simulink model "PIDPlus_1"  (R2023b)
settings: Solver=VariableStepAuto  StartTime=0.0  StopTime=50  RelTol=1e-3
undefined symbols (not defined in the file): Kd, Ki, Kp, Treset
settings Model: Creator=CANER  LastModifiedBy=CANER

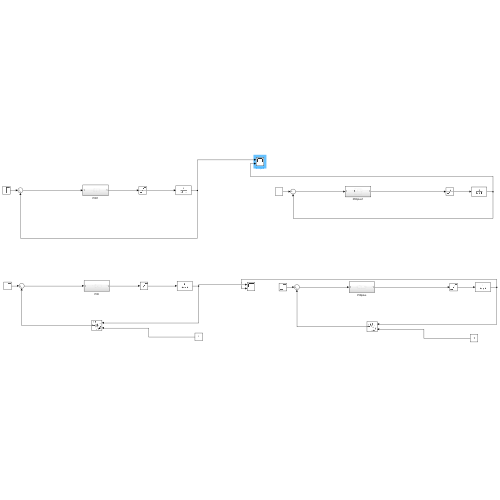
[thumbnail: Simulink's stored preview of the top-level diagram]
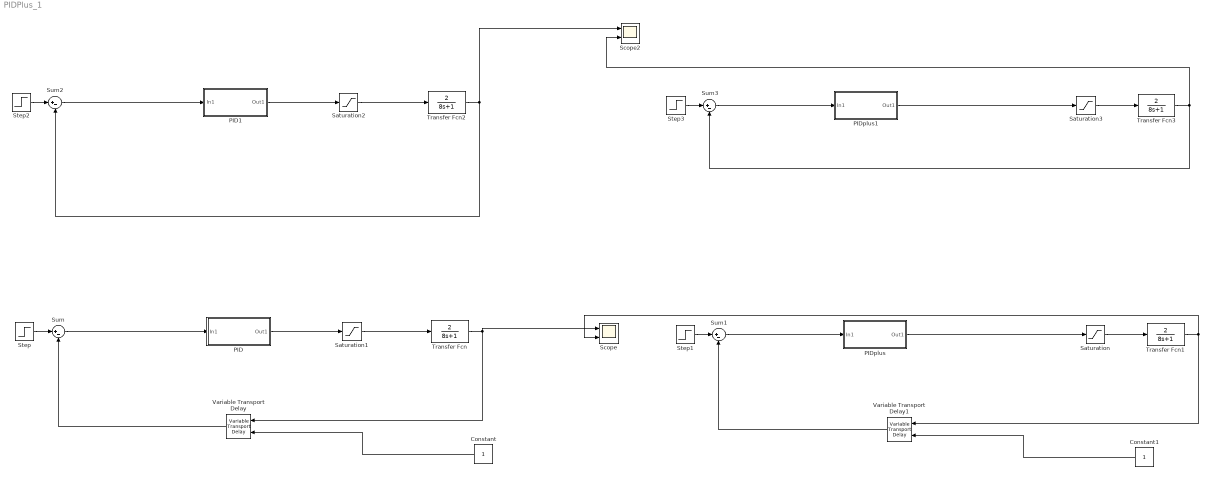
== system PIDPlus_1 ==
  Constant : Constant
  Constant1 : Constant
  PID : Subsystem
  PID1 : Subsystem
  PIDplus : Subsystem
  PIDplus1 : Subsystem
  Saturation{,1..3} (4 alike) : Saturate
  Scope : Scope  NumInputPorts=2
  Scope2 : Scope  NumInputPorts=2
  Step{,1..3} (4 alike) : Step  SampleTime=0
  Sum{,1..3} (4 alike) : Sum  Inputs=|+-
  Transfer Fcn{,1..3} (4 alike) : TransferFcn  Numerator=[2]  Denominator=[8 1]
  Variable Transport Delay : VariableTransportDelay  VariableDelayType=Variable transport delay  MaximumDelay=10
  Variable Transport Delay1 : VariableTransportDelay  VariableDelayType=Variable transport delay  MaximumDelay=10
  wires:
  Transfer Fcn/1 -> Scope/1, Variable Transport Delay/1
  Step/1 -> Sum/1
  Variable Transport Delay/1 -> Sum/2
  Constant/1 -> Variable Transport Delay/2
  Sum/1 -> PID/1(In1)
  PID/1(Out1) -> Saturation1/1
  Variable Transport Delay1/1 -> Sum1/2
  Transfer Fcn1/1 -> Scope/2, Variable Transport Delay1/1
  Constant1/1 -> Variable Transport Delay1/2
  Step1/1 -> Sum1/1
  Saturation/1 -> Transfer Fcn1/1
  Saturation1/1 -> Transfer Fcn/1
  Sum1/1 -> PIDplus/1(In1)
  PIDplus/1(Out1) -> Saturation/1
  PID1/1(Out1) -> Saturation2/1
  Saturation2/1 -> Transfer Fcn2/1
  Transfer Fcn2/1 -> Sum2/2, Scope2/1
  Sum2/1 -> PID1/1(In1)
  Step2/1 -> Sum2/1
  Sum3/1 -> PIDplus1/1(In1)
  Saturation3/1 -> Transfer Fcn3/1
  Step3/1 -> Sum3/1
  Transfer Fcn3/1 -> Sum3/2, Scope2/2
  PIDplus1/1(Out1) -> Saturation3/1

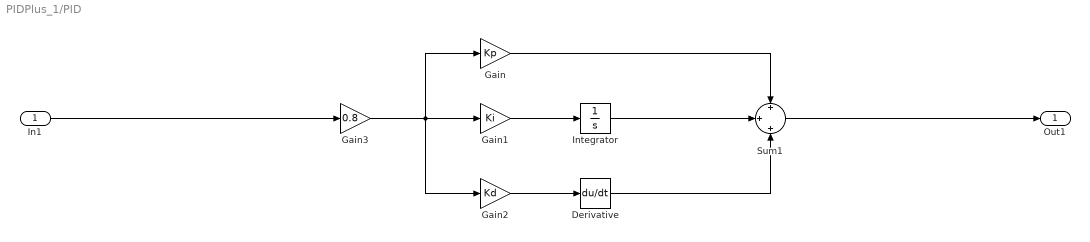
== system PIDPlus_1/PID ==
  In1 : Inport
  Derivative : Derivative
  Gain : Gain  Gain=Kp
  Gain1 : Gain  Gain=Ki
  Gain2 : Gain  Gain=Kd
  Gain3 : Gain  Gain=0.8
  Integrator : Integrator
  Sum1 : Sum  Inputs=+|+|+
  Out1 : Outport
  wires:
  In1/1 -> Gain3/1
  Sum1/1 -> Out1/1
  Integrator/1 -> Sum1/2
  Gain2/1 -> Derivative/1
  Gain/1 -> Sum1/1
  Gain1/1 -> Integrator/1
  Gain3/1 -> Gain2/1, Gain1/1, Gain/1
  Derivative/1 -> Sum1/3

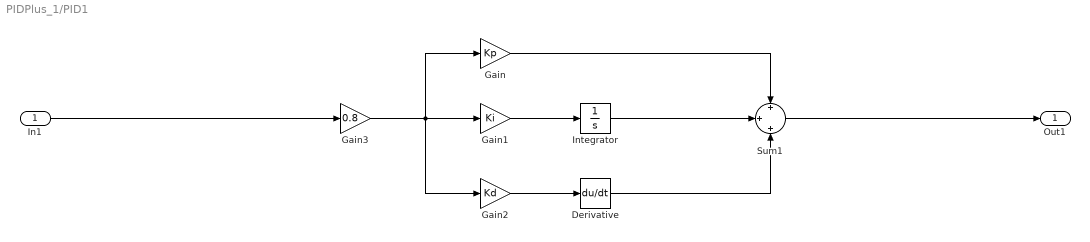
== system PIDPlus_1/PID1 ==
  In1 : Inport
  Derivative : Derivative
  Gain : Gain  Gain=Kp
  Gain1 : Gain  Gain=Ki
  Gain2 : Gain  Gain=Kd
  Gain3 : Gain  Gain=0.8
  Integrator : Integrator
  Sum1 : Sum  Inputs=+|+|+
  Out1 : Outport
  wires:
  In1/1 -> Gain3/1
  Sum1/1 -> Out1/1
  Integrator/1 -> Sum1/2
  Gain2/1 -> Derivative/1
  Gain/1 -> Sum1/1
  Gain1/1 -> Integrator/1
  Gain3/1 -> Gain2/1, Gain1/1, Gain/1
  Derivative/1 -> Sum1/3

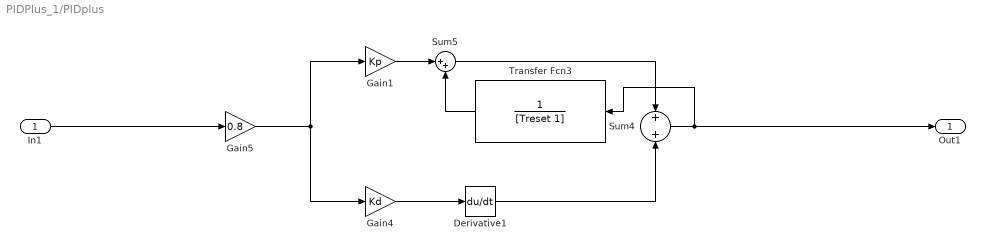
== system PIDPlus_1/PIDplus ==
  In1 : Inport
  Derivative1 : Derivative
  Gain1 : Gain  Gain=Kp
  Gain4 : Gain  Gain=Kd
  Gain5 : Gain  Gain=0.8
  Sum4 : Sum  Inputs=+|+
  Sum5 : Sum  Inputs=|++
  Transfer Fcn3 : TransferFcn  Denominator=[Treset 1]
  Out1 : Outport
  wires:
  Gain5/1 -> Gain4/1, Gain1/1
  Gain1/1 -> Sum5/1
  Gain4/1 -> Derivative1/1
  Sum4/1 -> Out1/1, Transfer Fcn3/1
  Derivative1/1 -> Sum4/2
  Transfer Fcn3/1 -> Sum5/2
  In1/1 -> Gain5/1
  Sum5/1 -> Sum4/1

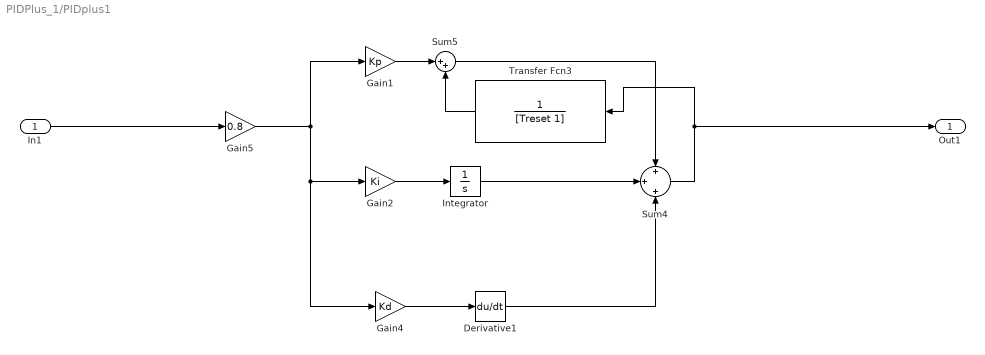
== system PIDPlus_1/PIDplus1 ==
  In1 : Inport
  Derivative1 : Derivative
  Gain1 : Gain  Gain=Kp
  Gain2 : Gain  Gain=Ki
  Gain4 : Gain  Gain=Kd
  Gain5 : Gain  Gain=0.8
  Integrator : Integrator
  Sum4 : Sum  Inputs=+|+|+
  Sum5 : Sum  Inputs=|++
  Transfer Fcn3 : TransferFcn  Denominator=[Treset 1]
  Out1 : Outport
  wires:
  Gain5/1 -> Gain2/1, Gain4/1, Gain1/1
  Gain1/1 -> Sum5/1
  Gain4/1 -> Derivative1/1
  Sum4/1 -> Out1/1, Transfer Fcn3/1
  Derivative1/1 -> Sum4/3
  Transfer Fcn3/1 -> Sum5/2
  In1/1 -> Gain5/1
  Sum5/1 -> Sum4/1
  Gain2/1 -> Integrator/1
  Integrator/1 -> Sum4/2
